simulink model "model_V2019b"  (R2023a)
settings: Solver=ode45  StartTime=0.0  StopTime=40  RelTol=1e-5  AbsTol=1e-5  EnableMultiTasking=on
undefined symbols (not defined in the file or in its folder): control, vr
settings Model: Creator=pmorin  LastModifiedBy=22044
settings SolverCC: AutoScaleAbsTol=off  AlgebraicLoopSolver=TrustRegion
settings DataIOCC: LimitDataPoints=on  SaveFormat=Array  SignalLoggingSaveFormat=ModelDataLogs  ReturnWorkspaceOutputs=off
settings OptimizationCC: BooleanDataType=off  ReuseModelBlockBuffer=off  ExpressionDepthLimit=2147483647  LifeSpan=inf
settings DebuggingCC: SaveWithParameterizedLinksMsg=none  UnderspecifiedInitializationDetection=Classic  MergeDetectMultiDrivingBlocksExec=none  SignalResolutionControl=TryResolveAllWithWarning  MultiTaskDSMMsg=warning  MultiTaskCondExecSysMsg=none  FcnCallInpInsideContextMsg=warning  UnconnectedInputMsg=warning  UnconnectedOutputMsg=warning  UnconnectedLineMsg=warning  StateNameClashWarn=warning  SFUnexpectedBacktrackingDiag=warning  SFNoUnconditionalDefaultTransitionDiag=warning  SFExecutionAtInitializationDiag=none  ArithmeticOperatorsInVariantConditions=warning
settings HardwareCC: ProdBitPerPointer=32  ProdBitPerSizeT=32  ProdBitPerPtrDiffT=32  ProdLargestAtomicFloat=None  ProdIntDivRoundTo=Undefined  ProdEndianess=Unspecified  ProdWordSize=32  ProdHWDeviceType=32-bit Generic  TargetUnknown=on
settings ModelReferenceCC: EnableRefExpFcnMdlSchedulingChecks=on  PropagateSignalLabelsOutOfModel=off
settings SFSimCC: SimUseLocalCustomCode=off  CustomCodeUndefinedFunction=UseInterfaceOnly
settings RTWCC: RTWUseLocalCustomCode=off
settings CodeAppCC: StateflowObjectComments=on
settings GRTTargetCC: TargetLangStandard=C89/C90 (ANSI)  CombineOutputUpdateFcns=off  GRTInterface=on
settings ConfigComp: CovMetricSettings=dw  CovSaveCumulativeToWorkspaceVar=on  CovSaveSingleToWorkspaceVar=on  CovExternalEMLEnable=off

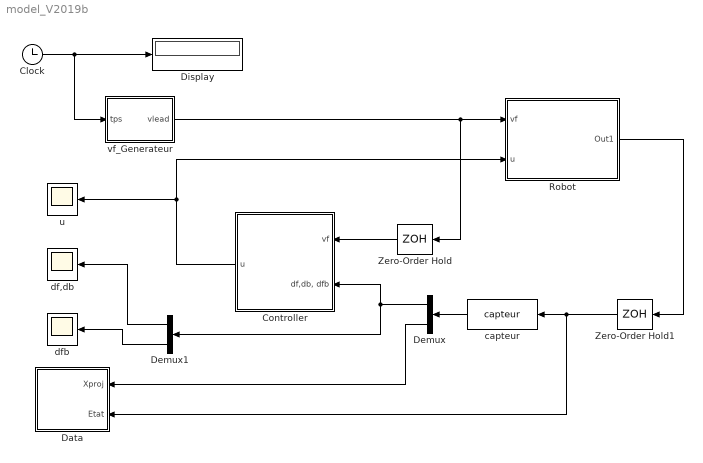
== system model_V2019b ==
  Clock : Clock
  Controller : Subsystem  mask{stomat=-1}
      mask prompts: stomat "Sample to matfile"
  Data : Subsystem  mask{stomat=-1}
      mask prompts: stomat "Sample to matfile"
  Demux : Demux  Outputs=[3;4]
  Demux1 : Demux  Outputs=[2;1]
  Display : Display
  Robot : Subsystem  mask{init=[2;8;0;2;4;-0.2]}
      mask prompts: init "Initial values"
  Zero-Order Hold : ZeroOrderHold  SampleTime=0.01
  Zero-Order Hold1 : ZeroOrderHold  SampleTime=0.01
  capteur : MATLABFcn  MATLABFcn=capteur  OutputDimensions=7
  df,db : Scope
  dfb : Scope
  u : Scope
  vf_Generateur : Subsystem  mask{choix_traj=vitesse quelconque}
      mask prompts: choix_traj "trajectoire de reference"
      mask TypeOptions choix_traj: vitesse positive | vitesse quelconque
  wires:
  Clock/1 -> vf_Generateur/1(tps), Display/1
  Controller/1(u) -> Robot/2(u), u/1
  vf_Generateur/1("vlead ") -> Zero-Order Hold/1, Robot/1(vf)
  Robot/1(Out1) -> Zero-Order Hold1/1
  Zero-Order Hold/1 -> Controller/1(vf)
  Zero-Order Hold1/1 -> Data/2(Etat), capteur/1
  capteur/1 -> Demux/1
  Demux/1 -> Demux1/1, Controller/2("df,db, dfb")
  Demux/2 -> Data/1(Xproj)
  Demux1/1 -> df,db/1
  Demux1/2 -> dfb/1

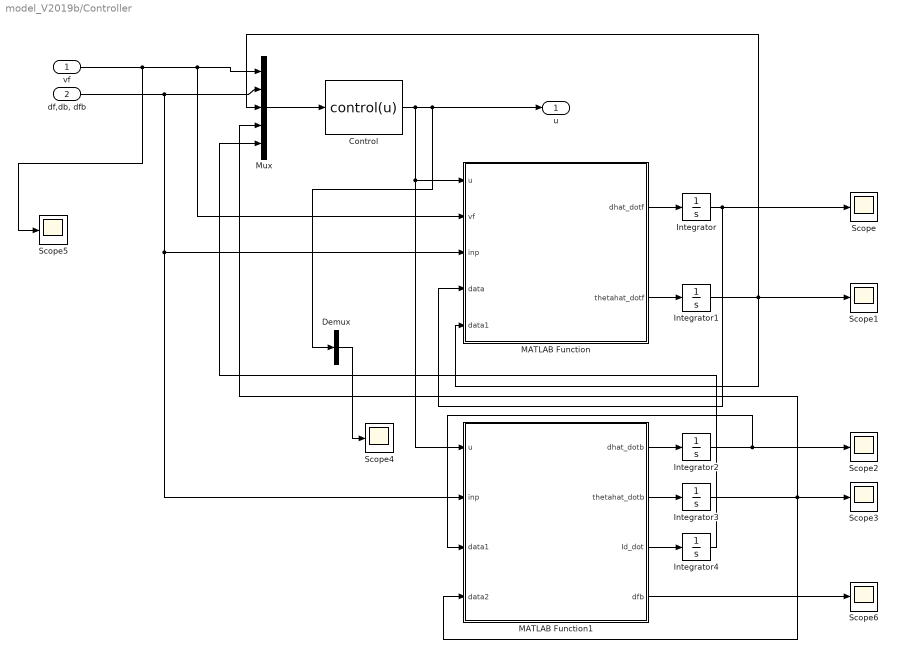
== system model_V2019b/Controller ==
  vf : Inport
  "df,db, dfb" : Inport  Port=2
  Control : MATLABFcn  MATLABFcn=control(u)  OutputDimensions=3
  Demux : Demux  Outputs=3
  Integrator{,1..4} (5 alike) : Integrator
  MATLAB Function : MATLAB Function  TreatAsAtomicUnit=on
  MATLAB Function1 : MATLAB Function  TreatAsAtomicUnit=on
  Mux : Mux  Inputs=5
  Scope{,1..6} (7 alike) : Scope
  u : Outport  VectorParamsAs1DForOutWhenUnconnected=off
  wires:
  Control/1 -> Demux/1, u/1, MATLAB Function1/1(u), MATLAB Function/1(u)
  vf/1 -> Scope5/1, MATLAB Function/2(vf), Mux/1
  "df,db, dfb"/1 -> MATLAB Function1/2(inp), MATLAB Function/3(inp), Mux/2
  Mux/1 -> Control/1
  MATLAB Function/1(dhat_dotf) -> Integrator/1
  Integrator/1 -> MATLAB Function/4(data), Scope/1
  MATLAB Function/2(thetahat_dotf) -> Integrator1/1
  Integrator1/1 -> MATLAB Function/5(data1), Mux/3, Scope1/1
  Integrator2/1 -> Scope2/1, MATLAB Function1/3(data1)
  Integrator3/1 -> MATLAB Function1/4(data2), Scope3/1, Mux/4
  MATLAB Function1/1(dhat_dotb) -> Integrator2/1
  MATLAB Function1/2(thetahat_dotb) -> Integrator3/1
  MATLAB Function1/3(Id_dot) -> Integrator4/1
  Integrator4/1 -> Mux/5
  MATLAB Function1/4(dfb) -> Scope6/1
  Demux/2 -> Scope4/1

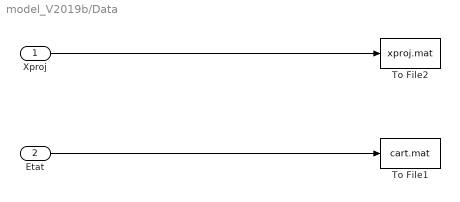
== system model_V2019b/Data ==
  Xproj : Inport
  Etat : Inport  Port=2
  To File1 : ToFile  Filename=cart.mat  SampleTime=stomat
  To File2 : ToFile  Filename=xproj.mat  SampleTime=stomat
  wires:
  Etat/1 -> To File1/1
  Xproj/1 -> To File2/1

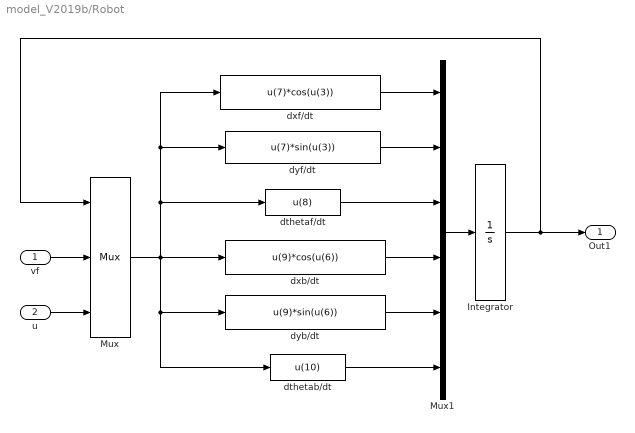
== system model_V2019b/Robot ==
  vf : Inport
  u : Inport  Port=2
  Integrator : Integrator  InitialCondition=init
  Mux : Mux  Inputs=[6 1 3]
  Mux1 : Mux  Inputs=6
  dthetab/dt : Fcn  Expr=u(10)
  dthetaf/dt : Fcn  Expr=u(8)
  dxb/dt : Fcn  Expr=u(9)*cos(u(6))
  dxf/dt : Fcn  Expr=u(7)*cos(u(3))
  dyb/dt : Fcn  Expr=u(9)*sin(u(6))
  dyf/dt : Fcn  Expr=u(7)*sin(u(3))
  Out1 : Outport  VectorParamsAs1DForOutWhenUnconnected=off
  wires:
  vf/1 -> Mux/2
  Integrator/1 -> Out1/1, Mux/1
  Mux1/1 -> Integrator/1
  dxf/dt/1 -> Mux1/1
  dyf/dt/1 -> Mux1/2
  dthetaf/dt/1 -> Mux1/3
  u/1 -> Mux/3
  dxb/dt/1 -> Mux1/4
  dyb/dt/1 -> Mux1/5
  Mux/1 -> dxf/dt/1, dyf/dt/1, dthetaf/dt/1, dthetab/dt/1, dyb/dt/1, dxb/dt/1
  dthetab/dt/1 -> Mux1/6

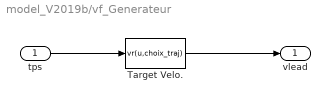
== system model_V2019b/vf_Generateur ==
  tps : Inport
  Target Velo. : MATLABFcn  MATLABFcn=vr(u,choix_traj)  OutputDimensions=1
  "vlead " : Outport  VectorParamsAs1DForOutWhenUnconnected=off
  wires:
  Target Velo./1 -> "vlead "/1
  tps/1 -> Target Velo./1

== matlab function model_V2019b/Controller/MATLAB Function1 ==
  data: u input; inp input; data1 input; data2 input; dhat_dotb output; thetahat_dotb output; Id_dot output; dfb output
function [dhat_dotb, thetahat_dotb, Id_dot,dfb] = fcn(u, inp, data1, data2)

% le veicule suiveur
u1=u(2);
u2=u(3);
dhatb=data1;
thetahatb=data2;
db=inp(2);
k1=0.5;
k2=0.5;

dhatdotb=u1*thetahatb - k1*abs(u1)*(dhatb-db);
thetahatdotb= u2 - k2*u1*(dhatb-db);

dhat_dotb= dhatdotb;
thetahat_dotb= thetahatdotb;
Id_dot=u1*db;

dfb=inp(3);

== matlab function model_V2019b/Controller/MATLAB Function ==
  data: u input; vf input; inp input; dhat_dotf output; data input; thetahat_dotf output; data1 input
function [dhat_dotf, thetahat_dotf] = fcn(u, vf, inp, data, data1)


% le veicule leader
u1=vf;
u2=u(1);
df=inp(1);
dhatf=data;
thetahatf=data1;
k1=1;
k2=1;

dhatdotf=u1*thetahatf - k1*abs(u1)*(dhatf-df);
thetahatdotf= u2 - k2*u1*(dhatf-df);

dhat_dotf= dhatdotf;
thetahat_dotf= thetahatdotf;
